simulink model "System_Model_Hall"  (Simulink 7.6)
settings: Solver=ode15s  StartTime=0.0  StopTime=3  RelTol=1e-3
undefined symbols (not defined in the file): F, G, g, H, K, L0, m, magnitude, Q, R, Ts, u0, x01, x02, x03
libraries: fl_lib x16, nesl_utility x5, elec_lib x3
CloseFcn:
  | rtwprivate ssgencode ModelCloseRequest System_Model1
settings Model: Creator=Fodi  LastModifiedBy=Fodi

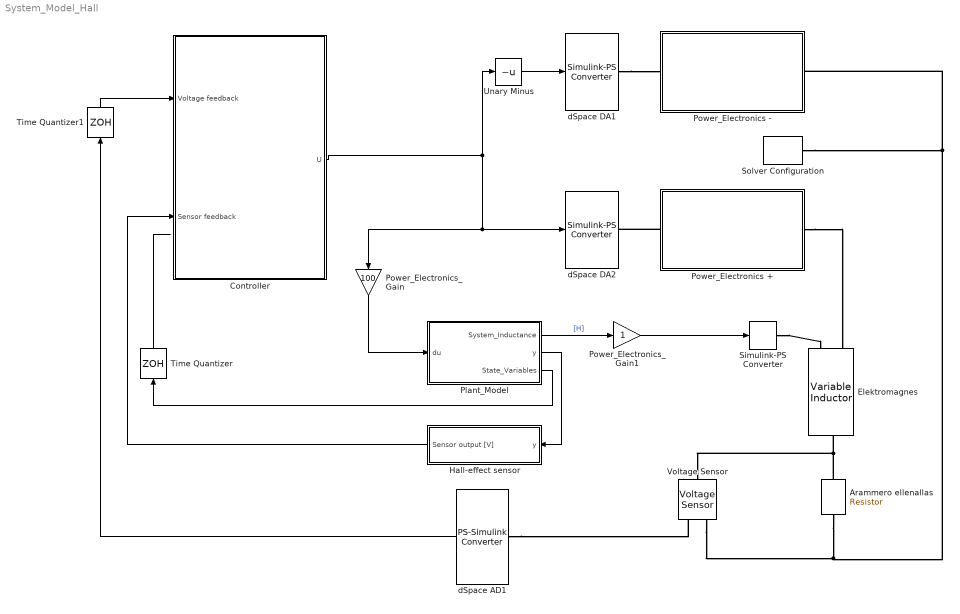
== system System_Model_Hall ==
  Arammero ellenallas : fl_lib/Electrical/Electrical Elements/Resistor  DialogController=NetworkEngine.DynNeDlgSource  SystemSampleTime=-1  R=30 Ohm  i_Log=off  v_Log=off  LocalVarNames=|i|v  LocalVarDescs=|i|v  LocalVarLogging=[0 0]
  Controller : Subsystem  TreatAsAtomicUnit=on  SystemSampleTime=Ts
  Elektromagnes : elec_lib/Passive Devices/Variable Inductor  DialogController=NetworkEngine.DynNeDlgSource  SystemSampleTime=-1  prm=2  Lmin=1e-6 H  g=1e-9 1/Ohm  i0=0 A  phi0=0 Wb  LocalVarLogging=[]
  Hall-effect sensor : Subsystem
  Plant_Model : Subsystem
  Power_Electronics + : Subsystem
  Power_Electronics - : Subsystem
  Power_Electronics_Gain : Gain  Gain=100
  Power_Electronics_Gain1 : Gain
  Simulink-PS Converter : nesl_utility/Simulink-PS Converter  DialogController=NetworkEngine.DynNeUtilDlgSource  SystemSampleTime=-1  PhysicalDomain=network_engine_domain  LeftPortType=input  RightPortType=output  SubClassName=ps_input  Unit=1  AffineConversion=off  InputFilterTimeConstant=.001  UdotUserProvided=0
  Solver Configuration : nesl_utility/Solver Configuration  DialogController=NetworkEngine.DynNeUtilDlgSource  SystemSampleTime=-1  PhysicalDomain=network_engine_domain  LeftPortType=input  RightPortType=generic  SubClassName=solver  Accelerate=off  Profile=off  ResidualTolerance=1e-9  MaxNonlinIter=3  MaxModeIter=2  DoFixedCost=off  UseLocalSampling=off  DoDC=off  LinearAlgebra=Sparse  LocalSolverSampleTime=.001  LocalSolverChoice=NE_BACKWARD_EULER_ADVANCER  UseLocalSolver=off
  Time Quantizer : ZeroOrderHold  SampleTime=Ts
  Time Quantizer1 : ZeroOrderHold  SampleTime=0.001
  Unary Minus : UnaryMinus
  Voltage Sensor : fl_lib/Electrical/Electrical Sensors/Voltage Sensor  DialogController=NetworkEngine.DynNeDlgSource  SystemSampleTime=-1  i1_Log=off  v1_Log=off  LocalVarNames=|i1|v1  LocalVarDescs=|i1|v1  LocalVarLogging=[0 0]
  dSpace AD1 : nesl_utility/PS-Simulink Converter  DialogController=NetworkEngine.DynNeUtilDlgSource  SystemSampleTime=-1  PhysicalDomain=network_engine_domain  LeftPortType=input  RightPortType=output  SubClassName=ps_output  Unit=1  AffineConversion=off
  dSpace DA1 : nesl_utility/Simulink-PS Converter  DialogController=NetworkEngine.DynNeUtilDlgSource  SystemSampleTime=-1  PhysicalDomain=network_engine_domain  LeftPortType=input  RightPortType=output  SubClassName=ps_input  Unit=1  AffineConversion=off  InputFilterTimeConstant=.001  UdotUserProvided=0
  dSpace DA2 : nesl_utility/Simulink-PS Converter  DialogController=NetworkEngine.DynNeUtilDlgSource  SystemSampleTime=-1  PhysicalDomain=network_engine_domain  LeftPortType=input  RightPortType=output  SubClassName=ps_input  Unit=1  AffineConversion=off  InputFilterTimeConstant=.001  UdotUserProvided=0
  wires:
  Plant_Model/1(System_Inductance) -> Power_Electronics_Gain1/1  "[H]"
  Power_Electronics_Gain/1 -> Plant_Model/1(du)
  Plant_Model/3(State_Variables) -> Time Quantizer/1
  Time Quantizer/1 -> ?
  Unary Minus/1 -> dSpace DA1/1
  Power_Electronics_Gain1/1 -> Simulink-PS Converter/1
  Controller/1(U) -> Unary Minus/1, dSpace DA2/1, Power_Electronics_Gain/1
  Time Quantizer1/1 -> Controller/1(Voltage feedback)
  dSpace AD1/1 -> Time Quantizer1/1
  Hall-effect sensor/1(Sensor output [V]) -> Controller/2(Sensor feedback)
  Plant_Model/2(y) -> Hall-effect sensor/1(y)
  connections:
  Power_Electronics +/LConn1 -- dSpace DA2/RConn1
  Arammero ellenallas/RConn1 -- Voltage Sensor/RConn2 -- Power_Electronics -/RConn1 -- Solver Configuration/RConn1
  Power_Electronics +/RConn1 -- Elektromagnes/LConn2
  Arammero ellenallas/LConn1 -- Elektromagnes/RConn1 -- Voltage Sensor/LConn1
  dSpace DA1/RConn1 -- Power_Electronics -/LConn1
  Simulink-PS Converter/RConn1 -- Elektromagnes/LConn1
  dSpace AD1/LConn1 -- Voltage Sensor/RConn1

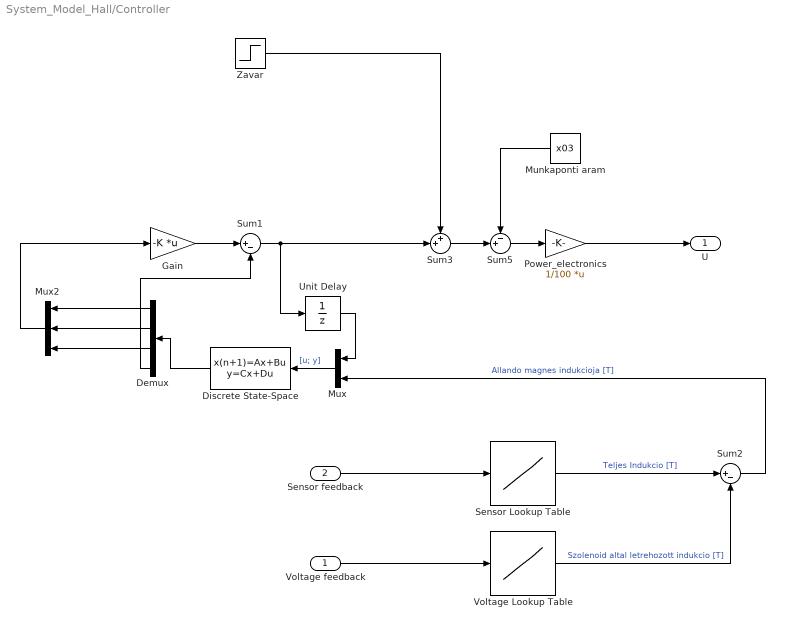
== system System_Model_Hall/Controller ==
  Voltage feedback : Inport
  Sensor feedback : Inport  Port=2
  Demux : Demux
  Discrete State-Space : DiscreteStateSpace  A=F  B=[H G]  C=eye(size(F))  D=zeros(size(F,1),size([H G],2))  SampleTime=Ts
  Gain : Gain  Gain=-K  Multiplication=Matrix(K*u)
  Munkaponti aram : Constant  Value=x03
  Mux : Mux  Inputs=2
  Mux2 : Mux  Inputs=3
  Power_electronics : Gain  Gain=1/100  Multiplication=Matrix(K*u)
  Sensor Lookup Table : Lookup  InputValues=[-5:5]  Table=tanh([-5:5])
  Sum1 : Sum  Inputs=|+-
  Sum2 : Sum  Inputs=|+-
  Sum3 : Sum  Inputs=++|
  Sum5 : Sum  Inputs=-+|
  Unit Delay : UnitDelay  SampleTime=-1
  Voltage Lookup Table : Lookup  InputValues=[-5:5]  Table=tanh([-5:5])
  Zavar : Step  Time=2  After=0  SampleTime=Ts
  U : Outport
  wires:
  Sum1/1 -> Unit Delay/1, Sum3/2
  Mux/1 -> Discrete State-Space/1  "[u; y]"
  Zavar/1 -> Sum3/1
  Mux2/1 -> Gain/1
  Demux/1 -> Mux2/1
  Discrete State-Space/1 -> Demux/1
  Unit Delay/1 -> Mux/1
  Munkaponti aram/1 -> Sum5/1
  Sum5/1 -> Power_electronics/1
  Sum3/1 -> Sum5/2
  Gain/1 -> Sum1/1
  Power_electronics/1 -> U/1
  Demux/2 -> Mux2/2
  Demux/3 -> Mux2/3
  Demux/4 -> Sum1/2
  Sensor feedback/1 -> Sensor Lookup Table/1
  Voltage feedback/1 -> Voltage Lookup Table/1
  Sensor Lookup Table/1 -> Sum2/1  "Teljes Indukcio [T]"
  Voltage Lookup Table/1 -> Sum2/2  "Szolenoid altal letrehozott indukcio [T]"
  Sum2/1 -> Mux/2  "Allando magnes indukcioja [T]"

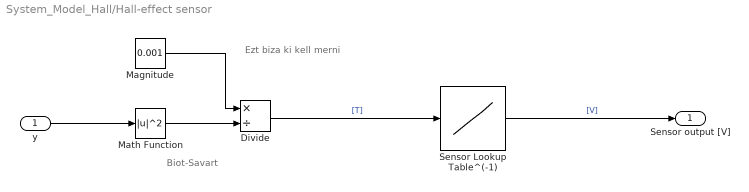
== system System_Model_Hall/Hall-effect sensor ==
  note: Ezt biza ki kell merni
  note: Biot-Savart
  y : Inport
  Divide : Product  Inputs=*/
  Magnitude : Constant  Value=0.001
  Math Function : Math  Operator=magnitude^2  SaturateOnIntegerOverflow=on
  Sensor Lookup Table^(-1) : Lookup  InputValues=[-5:5]  Table=tanh([-5:5])
  Sensor output [V] : Outport
  wires:
  y/1 -> Math Function/1
  Magnitude/1 -> Divide/1
  Math Function/1 -> Divide/2
  Divide/1 -> Sensor Lookup Table^(-1)/1  "[T]"
  Sensor Lookup Table^(-1)/1 -> Sensor output [V]/1  "[V]"

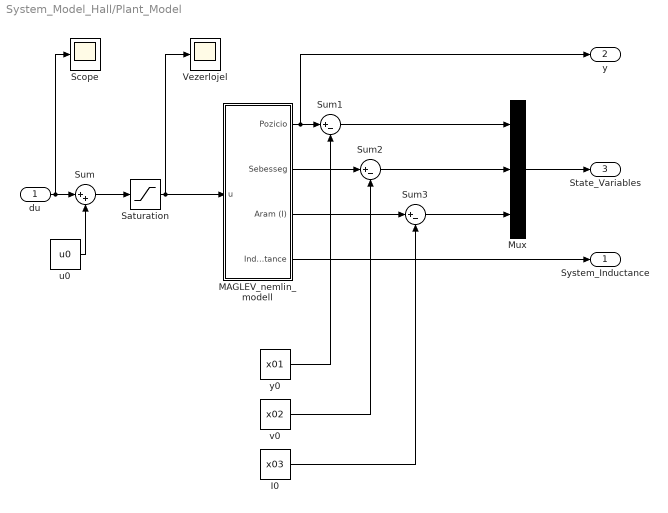
== system System_Model_Hall/Plant_Model ==
  du : Inport
  I0 : Constant  Value=x03
  MAGLEV_nemlin_modell : Subsystem
  Mux : Mux  Inputs=3
  Saturation : Saturate  UpperLimit=30  LowerLimit=-30
  Scope : Scope
  Sum : Sum  Inputs=|++
  Sum1 : Sum  Inputs=|+-
  Sum2 : Sum  Inputs=|+-
  Sum3 : Sum  Inputs=|+-
  Vezerlojel : Scope
      settings: TimeRange=10  YMin=11  YMax=16
  u0 : Constant  Value=u0
  v0 : Constant  Value=x02
  y0 : Constant  Value=x01
  System_Inductance : Outport
  y : Outport  Port=2
  State_Variables : Outport  Port=3
  wires:
  y0/1 -> Sum1/2
  v0/1 -> Sum2/2
  I0/1 -> Sum3/2
  MAGLEV_nemlin_modell/3(Aram (I)) -> Sum3/1
  Sum3/1 -> Mux/3
  Sum2/1 -> Mux/2
  Sum1/1 -> Mux/1
  u0/1 -> Sum/2
  Mux/1 -> State_Variables/1
  MAGLEV_nemlin_modell/2(Sebesseg) -> Sum2/1
  MAGLEV_nemlin_modell/1(Pozicio) -> Sum1/1, y/1
  du/1 -> Scope/1, Sum/1
  Sum/1 -> Saturation/1
  Saturation/1 -> MAGLEV_nemlin_modell/1(u), Vezerlojel/1
  MAGLEV_nemlin_modell/4(Inductance) -> System_Inductance/1

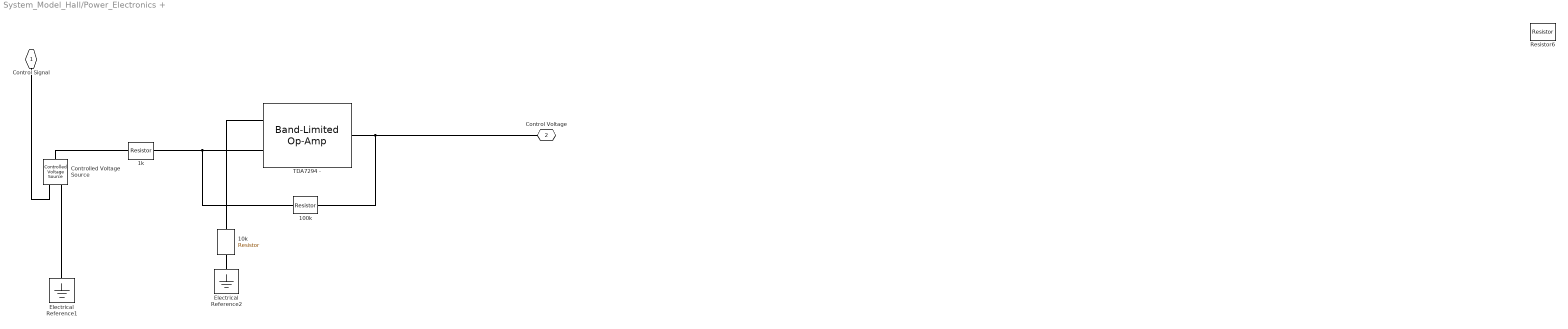
== system System_Model_Hall/Power_Electronics + ==
  100k : fl_lib/Electrical/Electrical Elements/Resistor  DialogController=NetworkEngine.DynNeDlgSource  SystemSampleTime=-1  R=10 kOhm  i_Log=off  v_Log=off  LocalVarNames=|i|v  LocalVarDescs=|i|v  LocalVarLogging=[0 0]
  10k : fl_lib/Electrical/Electrical Elements/Resistor  DialogController=NetworkEngine.DynNeDlgSource  SystemSampleTime=-1  R=100 kOhm  i_Log=off  v_Log=off  LocalVarNames=|i|v  LocalVarDescs=|i|v  LocalVarLogging=[0 0]
  1k : fl_lib/Electrical/Electrical Elements/Resistor  DialogController=NetworkEngine.DynNeDlgSource  SystemSampleTime=-1  R=100 Ohm  i_Log=off  v_Log=off  LocalVarNames=|i|v  LocalVarDescs=|i|v  LocalVarLogging=[0 0]
  Controlled Voltage Source : fl_lib/Electrical/Electrical Sources/Controlled Voltage Source  DialogController=NetworkEngine.DynNeDlgSource  SystemSampleTime=-1  i_Log=off  v_Log=off  LocalVarNames=|i|v  LocalVarDescs=|i|v  LocalVarLogging=[0 0]
  Electrical Reference1 : fl_lib/Electrical/Electrical Elements/Electrical Reference  DialogController=NetworkEngine.DynNeDlgSource  SystemSampleTime=-1  i_Log=off  LocalVarNames=|i  LocalVarDescs=|i  LocalVarLogging=0
  Electrical Reference2 : fl_lib/Electrical/Electrical Elements/Electrical Reference  DialogController=NetworkEngine.DynNeDlgSource  SystemSampleTime=-1  i_Log=off  LocalVarNames=|i  LocalVarDescs=|i  LocalVarLogging=0
  Resistor6 : fl_lib/Electrical/Electrical Elements/Resistor  DialogController=NetworkEngine.DynNeDlgSource  SystemSampleTime=-1  R=1 kOhm  i_Log=off  v_Log=off  LocalVarNames=|i|v  LocalVarDescs=|i|v  LocalVarLogging=[0 0]
  TDA7294 - : elec_lib/Integrated Circuits/Band-Limited Op-Amp  DialogController=NetworkEngine.DynNeDlgSource  SystemSampleTime=-1  A=10000  Rin=100 kOhm  Rout=100 Ohm  Vmin=-35 V  Vmax=35 V  Vdotmax=7000000 V/s  f=1e+5 Hz  V0=0 V  LocalVarLogging=[]
  Control Signal : PMIOPort  Tag=PMCPort  Port=1  Side=Left
  Control Voltage : PMIOPort  Tag=PMCPort  Port=2  Side=Right
  connections:
  1k/RConn1 -- TDA7294 -/LConn2 -- 100k/LConn1
  Electrical Reference1/LConn1 -- Controlled Voltage Source/RConn2
  Control Signal/RConn1 -- Controlled Voltage Source/RConn1
  10k/RConn1 -- Electrical Reference2/LConn1
  Control Voltage/RConn1 -- TDA7294 -/RConn1 -- 100k/RConn1
  TDA7294 -/LConn1 -- 10k/LConn1
  Controlled Voltage Source/LConn1 -- 1k/LConn1

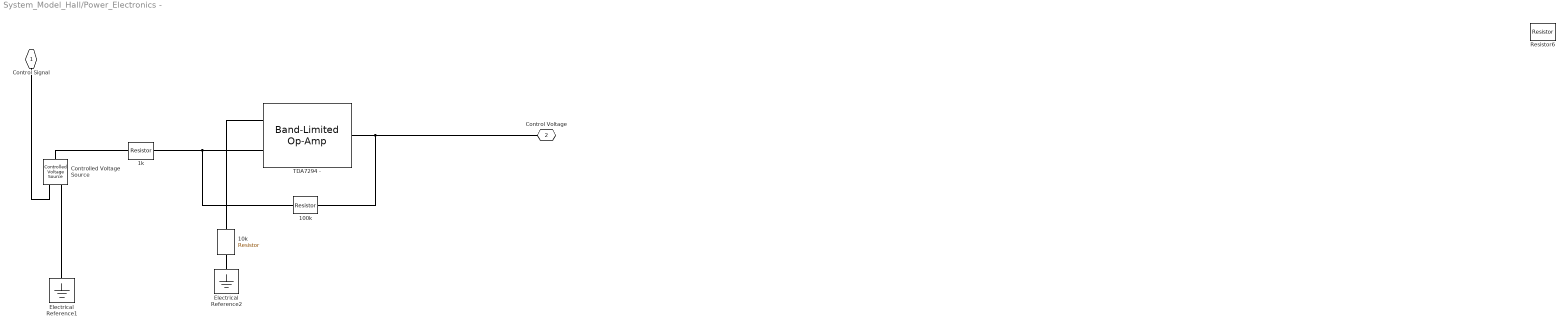
== system System_Model_Hall/Power_Electronics - ==
  100k : fl_lib/Electrical/Electrical Elements/Resistor  DialogController=NetworkEngine.DynNeDlgSource  SystemSampleTime=-1  R=100 kOhm  i_Log=off  v_Log=off  LocalVarNames=|i|v  LocalVarDescs=|i|v  LocalVarLogging=[0 0]
  10k : fl_lib/Electrical/Electrical Elements/Resistor  DialogController=NetworkEngine.DynNeDlgSource  SystemSampleTime=-1  R=10 kOhm  i_Log=off  v_Log=off  LocalVarNames=|i|v  LocalVarDescs=|i|v  LocalVarLogging=[0 0]
  1k : fl_lib/Electrical/Electrical Elements/Resistor  DialogController=NetworkEngine.DynNeDlgSource  SystemSampleTime=-1  R=1 kOhm  i_Log=off  v_Log=off  LocalVarNames=|i|v  LocalVarDescs=|i|v  LocalVarLogging=[0 0]
  Controlled Voltage Source : fl_lib/Electrical/Electrical Sources/Controlled Voltage Source  DialogController=NetworkEngine.DynNeDlgSource  SystemSampleTime=-1  i_Log=off  v_Log=off  LocalVarNames=|i|v  LocalVarDescs=|i|v  LocalVarLogging=[0 0]
  Electrical Reference1 : fl_lib/Electrical/Electrical Elements/Electrical Reference  DialogController=NetworkEngine.DynNeDlgSource  SystemSampleTime=-1  i_Log=off  LocalVarNames=|i  LocalVarDescs=|i  LocalVarLogging=0
  Electrical Reference2 : fl_lib/Electrical/Electrical Elements/Electrical Reference  DialogController=NetworkEngine.DynNeDlgSource  SystemSampleTime=-1  i_Log=off  LocalVarNames=|i  LocalVarDescs=|i  LocalVarLogging=0
  Resistor6 : fl_lib/Electrical/Electrical Elements/Resistor  DialogController=NetworkEngine.DynNeDlgSource  SystemSampleTime=-1  R=1 kOhm  i_Log=off  v_Log=off  LocalVarNames=|i|v  LocalVarDescs=|i|v  LocalVarLogging=[0 0]
  TDA7294 - : elec_lib/Integrated Circuits/Band-Limited Op-Amp  DialogController=NetworkEngine.DynNeDlgSource  SystemSampleTime=-1  A=10000  Rin=100 kOhm  Rout=100 Ohm  Vmin=-35 V  Vmax=35 V  Vdotmax=7000000 V/s  f=1e+5 Hz  V0=0 V  LocalVarLogging=[]
  Control Signal : PMIOPort  Tag=PMCPort  Port=1  Side=Left
  Control Voltage : PMIOPort  Tag=PMCPort  Port=2  Side=Right
  connections:
  Controlled Voltage Source/LConn1 -- 1k/LConn1
  TDA7294 -/LConn1 -- 10k/LConn1
  Control Voltage/RConn1 -- 100k/RConn1 -- TDA7294 -/RConn1
  10k/RConn1 -- Electrical Reference2/LConn1
  Control Signal/RConn1 -- Controlled Voltage Source/RConn1
  Electrical Reference1/LConn1 -- Controlled Voltage Source/RConn2
  100k/LConn1 -- TDA7294 -/LConn2 -- 1k/RConn1

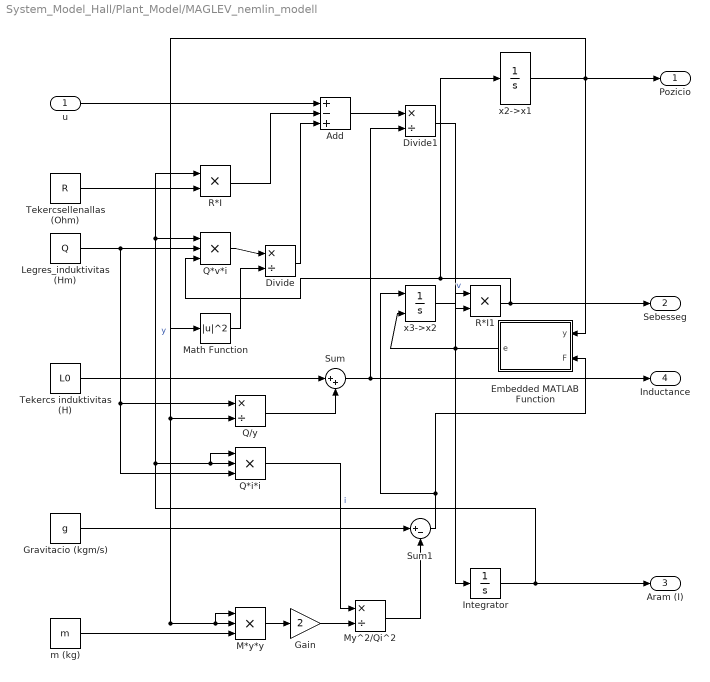
== system System_Model_Hall/Plant_Model/MAGLEV_nemlin_modell ==
  u : Inport  Tag=v
  Add : Sum  Inputs=+-+
  Divide : Product  Inputs=*/
  Divide1 : Product  Inputs=*/
  Embedded MATLAB Function : Stateflow chart  TreatAsAtomicUnit=on
  Gain : Gain  Gain=2
  Gravitacio (kgm/s) : Constant  Value=g
  Integrator : Integrator  InitialCondition=x03  LimitOutput=on  LowerSaturationLimit=0  ContinuousStateAttributes='current'
  Legres_induktivitas (Hm) : Constant  Value=Q
  M*y*y : Product  Inputs=3  RndMeth=Zero
  Math Function : Math  Operator=magnitude^2  SaturateOnIntegerOverflow=on
  My^2/Qi^2 : Product  Inputs=*/
  Q*i*i : Product  Inputs=3  RndMeth=Zero
  Q*v*i : Product  Inputs=3  RndMeth=Zero
  Q/y : Product  Inputs=*/
  R*I : Product  RndMeth=Zero
  R*I1 : Product  RndMeth=Zero
  Sum : Sum  Inputs=|++
  Sum1 : Sum  Inputs=|+-
  Tekercs induktivitas (H) : Constant  Value=L0
  Tekercsellenallas (Ohm) : Constant  Value=R
  m (kg) : Constant  Value=m
  x2->x1 : Integrator  InitialCondition=x01+0.001  LimitOutput=on  LowerSaturationLimit=0.001  ContinuousStateAttributes='position'
  x3->x2 : Integrator  ExternalReset=rising  ContinuousStateAttributes='speed'
  Pozicio : Outport
  Sebesseg : Outport  Port=2
  Aram (I) : Outport  Port=3
  Inductance : Outport  Port=4
  wires:
  x2->x1/1 -> Q/y/2, Math Function/1, M*y*y/2, M*y*y/1, Pozicio/1, Embedded MATLAB Function/1(y)  "y"
  Gravitacio (kgm/s)/1 -> Sum1/1
  My^2/Qi^2/1 -> Sum1/2
  Gain/1 -> My^2/Qi^2/2
  M*y*y/1 -> Gain/1
  Sum/1 -> Divide1/2, Inductance/1
  Tekercs induktivitas (H)/1 -> Sum/1
  Q/y/1 -> Sum/2
  Math Function/1 -> Divide/2
  Divide/1 -> Add/3
  Q*v*i/1 -> Divide/1
  R*I/1 -> Add/2
  Divide1/1 -> Integrator/1
  Add/1 -> Divide1/1
  u/1 -> Add/1
  m (kg)/1 -> M*y*y/3
  Legres_induktivitas (Hm)/1 -> Q*v*i/2, Q/y/1, Q*i*i/3
  Tekercsellenallas (Ohm)/1 -> R*I/2
  Q*i*i/1 -> My^2/Qi^2/1
  Integrator/1 -> Aram (I)/1, Q*i*i/2, Q*i*i/1, Q*v*i/1, R*I/1  "i"
  Sum1/1 -> x3->x2/1, Embedded MATLAB Function/2(F)
  Embedded MATLAB Function/1(e) -> x3->x2/2, R*I1/2
  R*I1/1 -> Q*v*i/3, x2->x1/1, Sebesseg/1
  x3->x2/1 -> R*I1/1  "v"

== matlab function Plant_Model/MAGLEV_nemlin_modell/Embedded MATLAB Function ==
  data: y input double; F input double; e output double
function e = fcn(y, F)
%#eml

if (F<=0 && y == 0.001)
    e=0;
else
    e=1;
end

end
